simulink model "composite_model"  (R2024a)
settings: Solver=FixedStepAuto  StartTime=0.0  StopTime=2  FixedStep=0.01  RelTol=1e-3
settings Model: Creator=amir  LastModifiedBy=amir

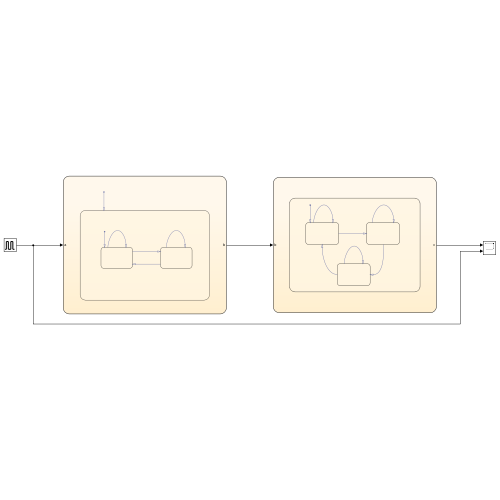
[thumbnail: Simulink's stored preview of the top-level diagram]
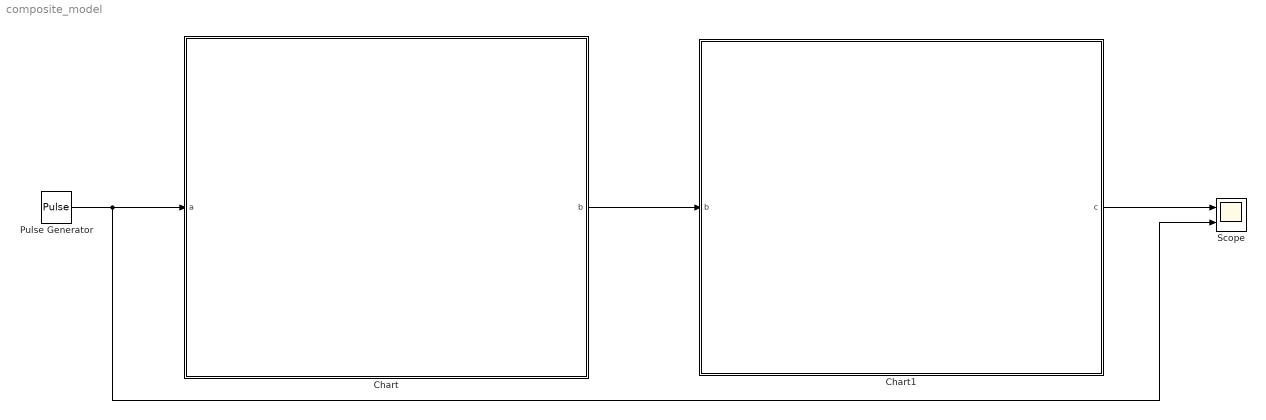
== system composite_model ==
  Chart : Stateflow chart  TreatAsAtomicUnit=on
  Chart1 : Stateflow chart  TreatAsAtomicUnit=on
  Pulse Generator : DiscretePulseGenerator  PulseType=Time based  Period=1  PulseWidth=6  PhaseDelay=0.05
  Scope : Scope  NumInputPorts=2
  wires:
  Pulse Generator/1 -> Scope/2, Chart/1(a)
  Chart/1(b) -> Chart1/1(b)
  Chart1/1(c) -> Scope/1

== stateflow chart composite_model/Chart1 ==
  state S2
    state X
    state Y
    state Z
    Y -> Y [order 2] : [~b]
    X -> X [order 2] : [~b]{c=0}
    (default) -> X
    X -> Y [order 1] : [b]{c=0}
    Z -> X [order 1] : [b]{c=1}
    Y -> Z [order 1] : [b]
    Z -> Z [order 2] : [~b]
  data: b input; c output

== stateflow chart composite_model/Chart ==
  state S1
    state A
    state B
    B -> B [order 2] : [~a]{b=0}
    A -> A [order 2] : [~a]{b=0}
    (default) -> A
    A -> B [order 1] : [a]{b=0}
    B -> A [order 1] : [a]{b=1}
  (default) -> S1 : {b=0;}
  data: a input; b output
